simulink model "simulink_discret"  (Simulink 8.4)
settings: Solver=ode45  StartTime=0.0  StopTime=25  MaxStep=0.001  RelTol=1e-3
values from neighbouring files (symbols this model uses):
  K_dis = acker(phi,gam,P_dis)    [Observador.m]    (also in P1.m; P1_pert.m; P1_pert_range.m; P1_pert_sin.m)
settings Model: Creator=student  LastModifiedBy=lluis
settings DebuggingCC: FcnCallInpInsideContextMsg=EnableAllAsWarning

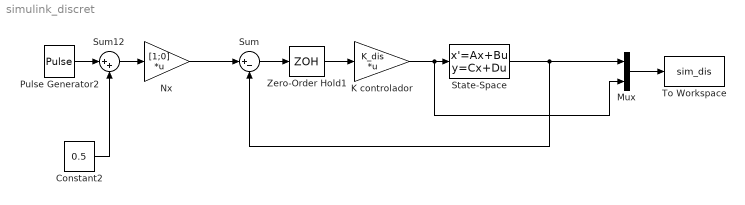
== system simulink_discret ==
  Constant2 : Constant  Value=0.5
  K controlador : Gain  Gain=K_dis  Multiplication=Matrix(K*u)
  Mux : Mux  Inputs=2
  Nx : Gain  Gain=[1;0]  Multiplication=Matrix(K*u)
  Pulse Generator2 : DiscretePulseGenerator  PulseType=Time based  Amplitude=-2  Period=20  PulseWidth=50
  State-Space : StateSpace  A=[0 -23.8095;0 0]  B=[0;-23.8095]  C=[1 0;0 1]  D=[0; 0]  X0=1
  Sum : Sum  Inputs=|+-
  Sum12 : Sum  Inputs=|++
  To Workspace : ToWorkspace  VariableName=sim_dis  SaveFormat=Timeseries  SampleTime=-1
  Zero-Order Hold1 : ZeroOrderHold  SampleTime=5E-2
  wires:
  State-Space/1 -> Sum/2, Mux/1
  Sum/1 -> Zero-Order Hold1/1
  Nx/1 -> Sum/1
  K controlador/1 -> State-Space/1, Mux/2
  Zero-Order Hold1/1 -> K controlador/1
  Mux/1 -> To Workspace/1
  Pulse Generator2/1 -> Sum12/1
  Constant2/1 -> Sum12/2
  Sum12/1 -> Nx/1
